simulink model "modele_cordeuse_veleves"  (R2015b)
settings: Solver=ode45  StartTime=0.0  StopTime=100  RelTol=1e-3
values from neighbouring files (symbols this model uses):
  eta = 29*55/(2*15)    (= 53.1666666667)    [para.m]
  Kd = 0    [para.m]
  Ke = 0.032    [para.m]
  Ki = 2000    [para.m]
  Kp = 1000    [para.m]
settings Model: Creator=David  LastModifiedBy=David
settings DataIOCC: SaveFormat=Array
settings DebuggingCC: SolverPrmCheckMsg=warning
settings HardwareCC: ProdBitPerPointer=32  ProdLargestAtomicFloat=None  ProdIntDivRoundTo=Undefined  ProdEndianess=Unspecified  ProdWordSize=32  ProdHWDeviceType=32-bit Generic
settings GRTTargetCC: GeneratePreprocessorConditionals=Disable all
settings ConfigComp: CovModelRefEnable=Off  CovSFcnEnable=off

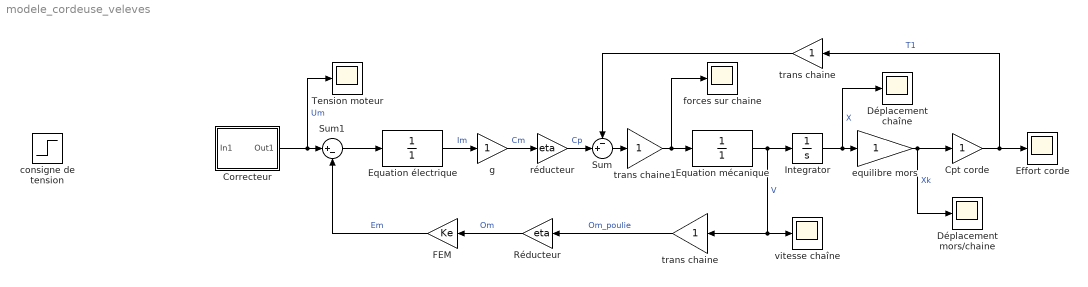
== system modele_cordeuse_veleves ==
  Correcteur : Subsystem
  Cpt corde : Gain
  Déplacement mors/chaine : Scope
  Déplacement chaîne : Scope
  Effort corde : Scope
  Equation mécanique : TransferFcn  Denominator=[1]
  Equation électrique : TransferFcn  Denominator=[1]
  FEM : Gain  Gain=Ke
  Integrator : Integrator
  Réducteur : Gain  Gain=eta
  Sum : Sum  Inputs=-+|
  Sum1 : Sum  Inputs=|+-
  Tension moteur : Scope
  consigne de tension : Step  After=100  SampleTime=0
  equilibre mors : Gain
  forces sur chaine : Scope
  "g " : Gain
  réducteur : Gain  Gain=eta
  trans chaine : Gain
  trans chaine1 : Gain
  trans chaine : Gain
  vitesse chaîne : Scope
  wires:
  Cpt corde/1 -> trans chaine/1, Effort corde/1  "T1"
  equilibre mors/1 -> Déplacement mors/chaine/1, Cpt corde/1  "Xk"
  Sum/1 -> trans chaine1/1
  Integrator/1 -> Déplacement chaîne/1, equilibre mors/1  "X"
  réducteur/1 -> Sum/2  "Cp"
  trans chaine/1 -> Sum/1
  "g "/1 -> réducteur/1  "Cm"
  Equation électrique/1 -> "g "/1  "Im"
  Sum1/1 -> Equation électrique/1
  Correcteur/1(Out1) -> Tension moteur/1, Sum1/1  "Um"
  FEM/1 -> Sum1/2  "Em"
  Equation mécanique/1 -> vitesse chaîne/1, trans chaine/1, Integrator/1  "V"
  Réducteur/1 -> FEM/1  "Om"
  trans chaine/1 -> Réducteur/1  "Om_poulie"
  trans chaine1/1 -> forces sur chaine/1, Equation mécanique/1

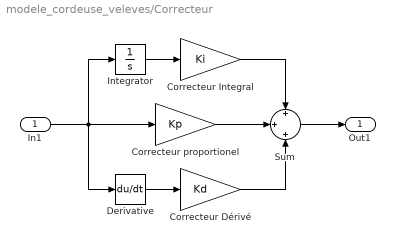
== system modele_cordeuse_veleves/Correcteur ==
  In1 : Inport
  Correcteur Dérivé : Gain  Gain=Kd
  Correcteur Integral : Gain  Gain=Ki
  Correcteur proportionel : Gain  Gain=Kp
  Derivative : Derivative
  Integrator : Integrator
  Sum : Sum  Inputs=+|+|+
  Out1 : Outport
  wires:
  In1/1 -> Derivative/1, Integrator/1, Correcteur proportionel/1
  Integrator/1 -> Correcteur Integral/1
  Correcteur Integral/1 -> Sum/1
  Correcteur proportionel/1 -> Sum/2
  Derivative/1 -> Correcteur Dérivé/1
  Correcteur Dérivé/1 -> Sum/3
  Sum/1 -> Out1/1
